simulink model "DSBSC generation"  (R2022b)
settings: Solver=VariableStepAuto  StartTime=0.0  StopTime=0.001  RelTol=1e-3
settings Model: Creator=mluser  LastModifiedBy=mluser

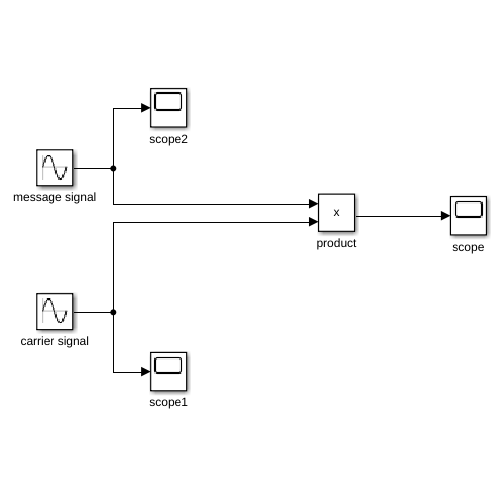
[thumbnail: Simulink's stored preview of the top-level diagram]
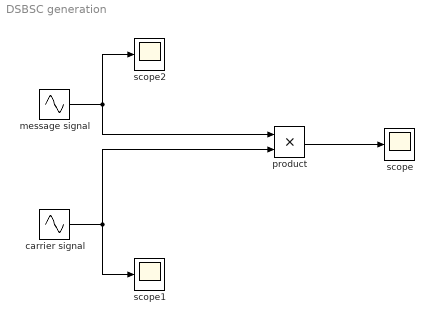
== system DSBSC generation ==
  carrier signal : Sin  Amplitude=3  Frequency=2*pi*50000  SampleTime=0
  message signal : Sin  Frequency=2*pi*2000  SampleTime=0
  product : Product
  scope : Scope
  scope1 : Scope
  scope2 : Scope
  wires:
  message signal/1 -> product/1, scope2/1
  carrier signal/1 -> product/2, scope1/1
  product/1 -> scope/1
